simulink model "linear_controller_PID_Feedforward"  (R2018a)
settings: Solver=VariableStepAuto  StartTime=0.0  StopTime=16  RelTol=1e-3
settings Model: Creator=ASUS  LastModifiedBy=ASUS

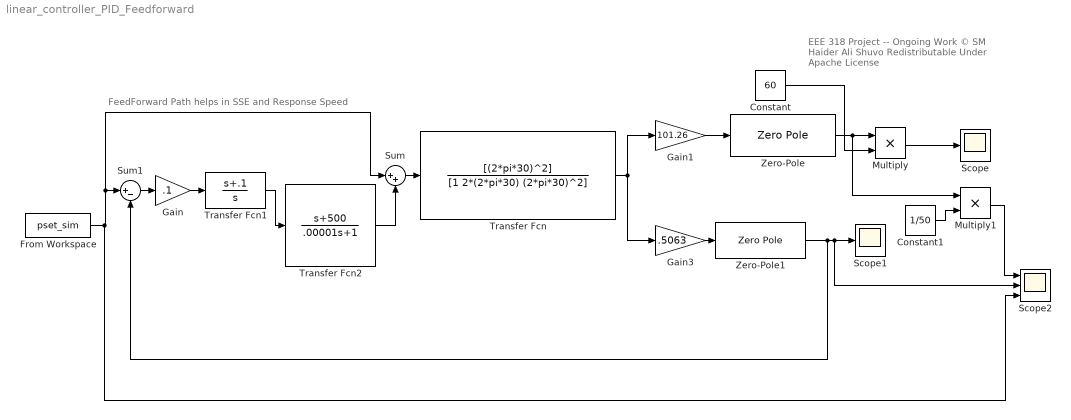
== system linear_controller_PID_Feedforward ==
  note: FeedForward Path helps in SSE and Response Speed
  note: EEE 318 Project -- Ongoing Work
      | © SM Haider Ali Shuvo
      | Redistributable Under Apache License
  Constant : Constant  Value=60
  Constant1 : Constant  Value=1/50
  From Workspace : FromWorkspace  VariableName=pset_sim  SampleTime=0
  Gain : Gain  Gain=.1
  Gain1 : Gain  Gain=101.26
  Gain3 : Gain  Gain=.5063
  Multiply : Product
  Multiply1 : Product
  Scope : Scope
  Scope1 : Scope
  Scope2 : Scope  NumInputPorts=3
  Sum : Sum  Inputs=|++
  Sum1 : Sum  Inputs=|+-
  Transfer Fcn : TransferFcn  Numerator=[(2*pi*30)^2]  Denominator=[1 2*(2*pi*30) (2*pi*30)^2]
  Transfer Fcn1 : TransferFcn  Numerator=[1 .1]  Denominator=[1 0]
  Transfer Fcn2 : TransferFcn  Numerator=[1 500]  Denominator=[.00001 1]
  Zero-Pole : ZeroPole  Zeros=[-8.88e-16]  Poles=[-5.4436]
  Zero-Pole1 : ZeroPole  Zeros=[-10]  Poles=[-5.4436]
  wires:
  Multiply/1 -> Scope/1
  Gain1/1 -> Zero-Pole/1
  Constant/1 -> Multiply/2
  Zero-Pole/1 -> Multiply1/1, Multiply/1
  From Workspace/1 -> Scope2/3, Sum/1, Sum1/1
  Zero-Pole1/1 -> Scope2/2, Scope1/1, Sum1/2
  Gain3/1 -> Zero-Pole1/1
  Sum1/1 -> Gain/1
  Transfer Fcn/1 -> Gain3/1, Gain1/1
  Gain/1 -> Transfer Fcn1/1
  Transfer Fcn1/1 -> Transfer Fcn2/1
  Transfer Fcn2/1 -> Sum/2
  Sum/1 -> Transfer Fcn/1
  Constant1/1 -> Multiply1/2
  Multiply1/1 -> Scope2/1
